simulink model "smo_pmsm"  (R2014a)
settings: Solver=ode45  StartTime=0.0  StopTime=3  RelTol=1e-3
PreLoadFcn:
  | parameter
InitFcn:
  | parameter
values from neighbouring files (symbols this model uses):
  R = 2e-3    (= 0.002)    [param.m]
undefined symbols (not defined in the file or in its folder): DiscIntNeverNeededParam, i_open_q, K, k_pll, ki_i, ki_pll, ki_v, kp_i, kp_pll, kp_v, L, sigbuilder_block, Threshold, TS, TS_time, upper, Vdc, wc, wc1, wc2
libraries: powerlib x4, AC6DriveInternalModels x1, simulink x1
Description:
  | parameter.m;
settings Model: SimulationMode=accelerator  Creator=jzj  LastModifiedBy=jzj
settings OptimizationCC: EfficientMapNaN2IntZero=off
settings HardwareCC: TargetLongLongMode=on  TargetIntDivRoundTo=Zero  TargetEndianess=LittleEndian  TargetHWDeviceType=MATLAB Host  ProdEqTarget=off
settings ModelReferenceCC: ModelDependencies=parameter.m;
settings CodeAppCC: MaxIdLength=128
settings GRTTargetCC: CombineOutputUpdateFcns=off  GRTInterface=on

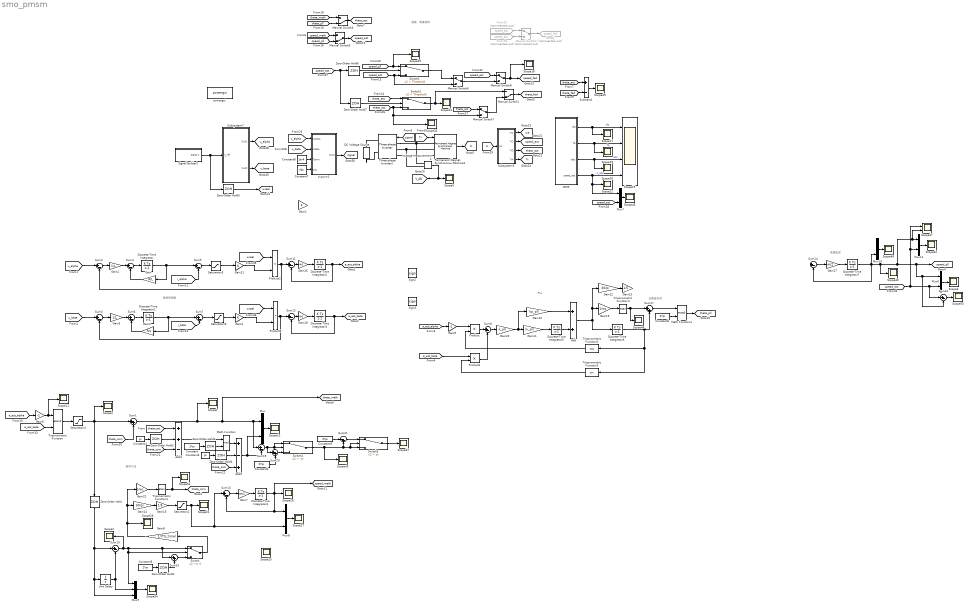
== system smo_pmsm ==
  note: 数学方法
  note: 滑模观测器
  note: 速度、角度选择
  note: 低通滤波
  note: PLL
  note: 加角度补偿
  Add : Sum
  Add1 : Sum  Inputs=++-
  Add2 : Sum  Inputs=+-+
  Constant{,2,5..6,9} (5 alike) : Constant  Value=2*pi
  Constant1 : Constant  Value=pi
  Constant3 : Constant  Value=pi
  Constant7 : Constant  Value=Vdc
  Constant8 : Constant  Value=1e-4
  DC Voltage Source : powerlib/Electrical Sources/DC Voltage Source  Amplitude=Vdc  Measurements=Voltage
  Discrete-Time Integrator{,1..3,6} (5 alike) : DiscreteIntegrator  SampleTime=-1  ICPrevOutput=DiscIntNeverNeededParam  ICPrevScaledInput=DiscIntNeverNeededParam
  Discrete-Time Integrator4 : DiscreteIntegrator  SampleTime=TS_time  ICPrevOutput=DiscIntNeverNeededParam  ICPrevScaledInput=DiscIntNeverNeededParam
  Discrete-Time Integrator5 : DiscreteIntegrator  InitialConditionSetting=State (most efficient)  SampleTime=-1  ICPrevOutput=DiscIntNeverNeededParam  ICPrevScaledInput=DiscIntNeverNeededParam
  Discrete-Time Integrator7 : DiscreteIntegrator  SampleTime=TS_time  ICPrevOutput=DiscIntNeverNeededParam  ICPrevScaledInput=DiscIntNeverNeededParam
  From15 : From  Commented=on  GotoTag=speed_act  TagVisibility=global
  From31 : From  Commented=on  GotoTag=speed_est  TagVisibility=global
  Gain : Gain  Gain=R/L
  Gain1 : Gain  Gain=K
  Gain10 : Gain  Gain=kp_pll
  Gain11 : Gain  Gain=ki_pll
  Gain12 : Gain  Gain=30/pi
  Gain13 : Gain  Gain=1/5
  Gain14 : Gain  Gain=30/pi
  Gain15 : Gain  Gain=1/5
  Gain16 : Gain  Gain=wc
  Gain17 : Gain  Gain=wc2
  Gain18 : Gain  Gain=wc
  Gain19 : Gain  Gain=1/wc
  Gain2 : Gain  Gain=1/L
  Gain20 : Gain  Gain=k_pll
  Gain21 : Gain  Gain=K
  Gain22 : Gain  Gain=2/wc
  Gain3 : Gain  Gain=R/L
  Gain4 : Gain  Gain=K
  Gain5 : Gain  Gain=1/L
  Gain6 : Gain  Gain=-1
  Gain7 : Gain  Gain=wc1
  Gain8 : Gain  Gain=1/(TS_time)
  Gain9 : Gain  Gain=-1
  Goto6 : Goto  Commented=on  GotoTag=speed_fed  TagVisibility=global
  Manual Switch1 : ManualSwitch  CurrentSetting=0
  Manual Switch2 : ManualSwitch  Commented=on
  Manual Switch3 : ManualSwitch  CurrentSetting=0
  Manual Switch5 : ManualSwitch  CurrentSetting=0
  Manual Switch6 : ManualSwitch
  Manual Switch7 : ManualSwitch
  Manual Switch8 : ManualSwitch
  Math Function : Math  Operator=mod  SaturateOnIntegerOverflow=on
  Math Function1 : Math  Operator=mod  SaturateOnIntegerOverflow=on
  Mux{,6..8,10..11} (6 alike) : Mux  Inputs=2
  Mux9 : Mux  Inputs=3
  Permanent Magnet Synchronous Machine1 : powerlib/Machines/Permanent Magnet Synchronous Machine  NbPhases=3  FluxDistribution=Sinusoidal  RotorType=Round  MechanicalLoad=Torque Tm  PresetModel=No  ShowDetailedParameters=on  MeasurementBus=off  Resistance=3  Inductance=0  dqInductances=[0.01,0.02]  La=0.0287  MachineConstant=Voltage Constant (V_peak L-L / krpm)  Flux=0.1654  VoltageCst=150  TorqueCst=1.2405  Flat=0  Mechanical=[0.001,0,5]  PolePairs=3  InitialConditions=[0,0, 0,0]  InitialConditions5ph=[0 0 0 0 0 0]  TsPowergui=0  TsBlock=-1  RefAngle=Aligned with phase A axis (original Park)
      link override From: GotoTag=tp24d3e2ed_e96a_4fb0_a076_5c3b1daf5e05
      settings: AttributesFormatString=\n
  Product{,1..3} (4 alike) : Product
  Saturation2 : Saturate  UpperLimit=5000  LowerLimit=-1000
  Saturation3 : Saturate  UpperLimit=upper  LowerLimit=-upper
  Saturation4 : Saturate  UpperLimit=pi  LowerLimit=-pi
  Saturation5 : Saturate  UpperLimit=upper  LowerLimit=-upper
  Scope{1..2,4..6,11,13,17..23,25..30,34,37,42..44,46,48..49,52,54..55} (31 alike) : Scope
      Scope1 settings: YMin=-700  YMax=700  SaveName=ScopeData7
      Scope11 settings: YMin=-700  YMax=700  SaveName=ScopeData25
      Scope13 settings: YMin=-700  YMax=700  SaveName=ScopeData32
      Scope17 settings: YMin=-700  YMax=700  SaveName=ScopeData18
      Scope18 settings: YMin=-700  YMax=700  SaveName=ScopeData35
      Scope19 settings: TimeRange=1.5  YMin=-700  YMax=700  SaveName=ScopeData19
      Scope2 settings: YMin=-700  YMax=700  SaveName=ScopeData10
      Scope20 settings: YMin=-0.04  YMax=0.04
      Scope21 settings: TimeRange=0.5  YMin=4000  YMax=4003  SaveName=ScopeData4
      Scope22 settings: YMin=-700  YMax=700  SaveName=ScopeData36
      Scope23 settings: YMin=-700  YMax=700  SaveName=ScopeData39
      Scope25 settings: YMin=-700  YMax=700  SaveName=ScopeData41
      Scope26 settings: YMin=-700  YMax=700  SaveName=ScopeData42
      Scope27 settings: YMin=-700  YMax=700  SaveName=ScopeData43
      Scope28 settings: YMin=-700  YMax=700  SaveName=ScopeData44
      Scope29 settings: YMin=-700  YMax=700  SaveName=ScopeData45
      Scope30 settings: YMin=-700  YMax=700  SaveName=ScopeData46
      Scope34 settings: YMin=-700  YMax=700  SaveName=ScopeData74
      Scope37 settings: YMin=-700  YMax=700  SaveName=ScopeData54
      Scope4 settings: YMin=-700  YMax=700  SaveName=ScopeData13
      Scope42 settings: YMin=-700  YMax=700  SaveName=ScopeData60
      Scope43 settings: YMin=-700  YMax=700  SaveName=ScopeData61
      Scope44 settings: YMin=-700  YMax=700  SaveName=ScopeData62
      Scope46 settings: TimeRange=0.5  YMin=0  YMax=600  SaveName=ScopeData63
      Scope48 settings: YMin=-700  YMax=700  SaveName=ScopeData73
      Scope49 settings: YMin=-700  YMax=700  SaveName=ScopeData80
      Scope5 settings: YMin=-700  YMax=700  SaveName=ScopeData78
      Scope52 settings: YMin=-700  YMax=700  SaveName=ScopeData77
      Scope54 settings: YMin=-700  YMax=700  SaveName=ScopeData81
      Scope55 settings: YMin=-700  YMax=700  SaveName=ScopeData85
      Scope6 settings: YMin=-700  YMax=700  SaveName=ScopeData14
  Scope15 : Scope  NumInputPorts=4
      settings: TimeRange=1.5  YMin=-17.5~-5~-80~-400  YMax=15~35~60~900  SaveName=ScopeData20
  Scope47 : Scope  NumInputPorts=2
      settings: YMin=-700~-5  YMax=700~5  SaveName=ScopeData76
  Sign2 : Signum
  Sign3 : Signum
  Signal Builder1 : Subsystem  Tag=STV Subsys  LoadFcn=sigbuilder_block('load');  StartFcn=sigbuilder_block('start');  StopFcn=sigbuilder_block('stop');  ClipboardFcn=sigbuilder_block('clipboard');  mask(Sigbuilder block){}
      mask help: Simulink:masks:SigbuilderBlock_MD
      mask init:
      | if ~strcmp(get_param(bdroot(gcbh),'SimulationStatus'),'stopped') tuvar = sigbuilder_block('maskInit'); end
      settings: CopyFcn=sigbuilder_block('copy');  DeleteFcn=sigbuilder_block('delete');  ModelCloseFcn=sigbuilder_block('modelClose');  PreSaveFcn=sigbuilder_block('preSave');  PauseFcn=sigbuilder_block('pause');  ContinueFcn=sigbuilder_block('continue');  NameChangeFcn=sigbuilder_block('namechange');  OpenFcn=sigbuilder_block('open',[6.75 -95.25 1138.5 566.25 ]);  CloseFcn=sigbuilder_block('close');
      mask Display: plot(0, 0, 100, 100,[2, 2, 32, 32, 2], [68, 8, 8, 68, 68],[32, 2], [38, 38], [32, 19, 2],[53, 60, 44], [32, 17, 17, 2],[16, 16, 31, 31]);txt = getActiveGroup(gcbh);text(2, 100, txt,'verticalAlignment', 'top');
  Subsystem3 : Subsystem
  Subsystem7 : Subsystem
  Subtract1 : Sum  Inputs=+-
  Sum{1,15,17,20} (4 alike) : Sum  Inputs=|++
  Sum{2..8,10..14,19,24} (14 alike) : Sum  Inputs=|+-
  Sum21 : Sum  Inputs=|-+
  Switch : Switch
  Switch1 : Switch  Criteria=u2 > Threshold  Threshold=Threshold
  Switch2 : Switch  Criteria=u2 > Threshold  Threshold=Threshold
  Switch4 : Switch  Criteria=u2 > Threshold  Threshold=-pi
  Switch5 : Switch  Criteria=u2 > Threshold  Threshold=pi
  Three-phase Inverter2 : AC6DriveInternalModels/Three-phase Inverter  Arms=3  SnubberResistance=5000  SnubberCapacitance=inf  Device=IGBT / Diodes  Ron=1e-3  Lon=0  ForwardVoltages=[0.8,0.8]  ForwardVoltage=0  GTOparameters=[0,0]  IGBTParameters=[1e-6,2e-6]  Measurements=All voltages and currents  converterType=Inverter  SourceFrequency=60  dqInductances=[8.5e-3,8.5e-3]  Flux=0.175  Resistance=0.2  p=4
  Trigonometric Function : Trigonometry  Operator=atan2
  Trigonometric Function1 : Trigonometry  Operator=atan
  Trigonometric Function2 : Trigonometry  Operator=cos
  Trigonometric Function3 : Trigonometry
  Trigonometric Function4 : Trigonometry  Operator=atan
  Unit Delay : UnitDelay  SampleTime=-1
  Voltage Measurement1 : powerlib/Measurements/Voltage Measurement  PhasorSimulation=off  OutputType=Complex  PSBequivalent=0
  Zero-Order Hold : ZeroOrderHold  SampleTime=TS_time
  Zero-Order Hold{1..7} (7 alike) : ZeroOrderHold  SampleTime=TS
  powergui : powerlib/powergui  Priority=1  SimulationMode=Discrete  SolverType=Tustin  SampleTime=1e-6  frequency=60  SPID=off  DisableSnubberDevices=off  DisableRonSwitches=off  DisableVfSwitches=off  SwTol=0  Interpol=off  DisplayEquations=off  Ts=100  methode=off  frequencyindice=0  Pbase=100e6  ErrMax=1e-4  Iterations=50  UnitsV=kV  UnitsW=MW  FunctionMessages=off  echomessages=off  HookPort=off  EnableUseOfTLC=off  x0status=blocks  RestoreLinks=warning  ResistiveCurrentMeasurement=off  Frange=[0:2:500]  Ylog=off  Xlog=on  ShowGrid=off  save=off  variable=ZData  structure=iabc1  ZoomFFT=off  StartTime=2.2  cycles=50  DisplayStyle=1  fundamental=200  FreqAxis=on  MaxFrequency=500  frequencyindicesteady=1  RmsSteady=1  display=off
  state : Subsystem
  svpwm1 : Subsystem
  tag scope: Tr=global, V_AB=global, e_est_alpha=global, e_est_beta=global, m=global, signal=global, speed_act=global, speed_est=global, speed_fed=global, speed_math=global, speed_pll=global, theta_act=global, theta_com=global, theta_est=global, theta_fed=global, theta_math=global, theta_pll=global, u_alpha=global, u_beta=global, we=global, wreal=global
  wires:
  Subsystem7/1(Out1) -> [u_alpha]
  Subsystem7/2(Out2) -> [u_beta]
  Constant8/1 -> svpwm1/3(Tpwm)
  Constant7/1 -> svpwm1/4(Vdc)
  svpwm1/1(Out1) -> [signal]
  [u_alpha] -> svpwm1/1(Valpha)
  [u_beta] -> svpwm1/2(Vbeta)
  [Tr] -> Permanent Magnet Synchronous Machine1/1
  Permanent Magnet Synchronous Machine1/1 -> [m]
  Voltage Measurement1/1 -> [V_AB], Scope5/1
  [m] -> Subsystem3/1(In1)
  Subsystem3/1(Tr1) -> [we]
  Subsystem3/2(Tr2) -> [speed_act]
  Subsystem3/3(Tr3) -> [theta_act]
  Subsystem3/4(Tr4) -> [Tr]
  state/1(idq) -> Scope17/1, Scope15/1  "idq"
  state/2(Te) -> Scope19/1, Scope15/2  "Te"
  state/3(iabc) -> Scope20/1, Scope15/3  "iabc"
  state/4(speed_obs) -> Mux7/1, Scope21/1, Scope15/4  "n_obs"
  Sum2/1 -> Gain2/1
  Sum4/1 -> Discrete-Time Integrator/1
  Gain/1 -> Sum4/2
  Discrete-Time Integrator/1 -> Sum5/1, Gain/1
  [i_alpha] -> Sum5/2
  Sum5/1 -> Saturation3/1
  Saturation3/1 -> Gain21/1
  Gain2/1 -> Sum4/1
  Sum6/1 -> Discrete-Time Integrator1/1
  Gain3/1 -> Sum6/2
  Discrete-Time Integrator1/1 -> Gain3/1, Sum7/1
  [i_beta] -> Sum7/2
  Sum7/1 -> Saturation5/1
  Saturation5/1 -> Gain4/1
  Gain5/1 -> Sum6/1
  Sum3/1 -> Gain5/1
  Gain6/1 -> Scope11/1, Trigonometric Function/1
  Product3/1 -> Sum3/2, Sum12/1
  Constant/1 -> Zero-Order Hold3/1
  Mux/1 -> Scope13/1
  [speed_act] -> Manual Switch6/2, Switch1/3
  [speed_pll] -> Scope29/1, Switch1/1
  [theta_est] -> Switch2/1
  [speed_est] -> Zero-Order Hold6/1, Zero-Order Hold7/1
  [theta_act] -> Switch2/3, Manual Switch7/2, Scope34/1
  Switch2/1 -> Scope23/1, Manual Switch1/1
  Trigonometric Function/1 -> Saturation4/1
  Gain8/1 -> Scope28/1, Gain14/1, Gain22/1
  Zero-Order Hold/1 -> Mux9/3, Unit Delay/1, Sum10/1
  Unit Delay/1 -> Sum10/2, Mux9/2
  Gain14/1 -> Gain15/1
  Sum11/1 -> Gain16/1
  Gain16/1 -> Discrete-Time Integrator2/1
  Discrete-Time Integrator2/1 -> [e_est_alpha], Sum11/2
  Sum12/1 -> Gain18/1
  Gain18/1 -> Discrete-Time Integrator3/1
  Discrete-Time Integrator3/1 -> [e_est_beta], Sum12/2
  Sum1/1 -> [theta_math], Sum19/1, Mux/1, Scope1/1
  Saturation4/1 -> Zero-Order Hold/1, Sum1/1, Scope4/1
  Gain15/1 -> Saturation2/1
  Mux9/1 -> Scope54/1
  Sum10/1 -> Scope2/1, Mux9/1, Switch/2, Sum15/1, Switch/1
  Sum15/1 -> Switch/3
  Switch/1 -> Gain8/1
  Sum13/1 -> Gain7/1
  Gain7/1 -> Discrete-Time Integrator4/1
  Discrete-Time Integrator4/1 -> [speed_math], Sum13/2, Mux8/1, Scope26/1
  Mux8/1 -> Scope27/1
  Manual Switch3/1 -> [theta_est]
  [e_est_alpha] -> Gain9/1
  Gain9/1 -> Product/1
  Product/1 -> Sum8/1
  Gain10/1 -> Add/1
  Discrete-Time Integrator5/1 -> Add/2
  Gain11/1 -> Discrete-Time Integrator5/1
  Sum8/1 -> Gain20/1
  Add/1 -> Gain19/1, Gain12/1, Discrete-Time Integrator6/1
  Discrete-Time Integrator6/1 -> Trigonometric Function3/1, Trigonometric Function2/1, Sum17/2
  Gain12/1 -> Gain13/1
  Trigonometric Function2/1 -> Product/2
  [e_est_beta] -> Product1/1
  Trigonometric Function3/1 -> Product1/2
  Product1/1 -> Sum8/2
  [theta_math] -> Manual Switch3/1
  [theta_pll] -> Manual Switch3/2
  Manual Switch5/1 -> [speed_est]
  [speed_math] -> Manual Switch5/1
  [speed_pll] -> Manual Switch5/2
  Sum14/1 -> Gain17/1
  Gain17/1 -> Discrete-Time Integrator7/1
  Discrete-Time Integrator7/1 -> Mux10/2, Sum14/2, Scope30/1, Scope47/2, Mux11/1, Sum24/2, Mux6/1, [speed_pll]
  Add1/1 -> Math Function/1
  Add2/1 -> Sum19/2, Mux/2
  Gain22/1 -> Trigonometric Function1/1
  Trigonometric Function1/1 -> Scope52/1, [theta_com]
  [theta_com] -> Sum1/2
  [theta_act] -> Add1/1
  Constant1/1 -> Zero-Order Hold2/1
  [theta_com] -> Add1/3
  Math Function/1 -> Add2/1
  Constant3/1 -> Zero-Order Hold4/1
  [theta_com] -> Add2/3
  Gain19/1 -> Trigonometric Function4/1
  Constant5/1 -> Zero-Order Hold1/1
  Zero-Order Hold2/1 -> Add1/2
  Zero-Order Hold3/1 -> Math Function/2
  Zero-Order Hold4/1 -> Add2/2
  Zero-Order Hold6/1 -> Switch1/2
  Zero-Order Hold7/1 -> Switch2/2
  Saturation2/1 -> Scope22/1, Sum13/1, Mux8/2
  Zero-Order Hold1/1 -> Sum15/2
  Gain20/1 -> Gain10/1, Gain11/1
  [speed_est] -> Mux7/2
  Mux7/1 -> Scope46/1
  Mux10/1 -> Scope48/1
  Signal Builder1/1(Signal 1) -> Zero-Order Hold5/1, Subsystem7/1(n_ref)
  [theta_act] -> Subtract1/1
  [theta_fed] -> Subtract1/2
  Subtract1/1 -> Scope49/1
  Manual Switch1/1 -> [theta_fed]
  From31/1 -> Manual Switch2/1
  From15/1 -> Manual Switch2/2
  Manual Switch2/1 -> Goto6/1
  Switch1/1 -> Manual Switch6/1
  [theta_act] -> Manual Switch7/1
  Manual Switch7/1 -> Manual Switch1/2
  Manual Switch6/1 -> Manual Switch8/2
  [speed_act] -> Manual Switch8/1
  Manual Switch8/1 -> Scope18/1, [speed_fed]
  [e_est_alpha] -> Gain6/1
  [e_est_beta] -> Trigonometric Function/2
  [u_alpha] -> Sum2/1
  [u_beta] -> Sum3/1
  [signal] -> Three-phase Inverter2/1
  Sum17/1 -> Math Function1/1
  Constant6/1 -> Math Function1/2
  Product2/1 -> Sum2/2, Sum11/1
  Sum19/1 -> Sum20/1, Switch4/1, Switch4/2
  Sum20/1 -> Switch4/3
  Constant2/1 -> Sum20/2
  Switch4/1 -> Scope43/1, Sum21/2, Switch5/2, Switch5/3
  Sum21/1 -> Switch5/1
  Constant9/1 -> Sum21/1
  Switch5/1 -> Scope37/1
  [speed_act] -> Scope47/1, Mux11/2, Sum24/1, Mux6/2
  Mux6/1 -> Scope6/1
  Mux11/1 -> Scope42/1
  Zero-Order Hold5/1 -> [wreal]
  Gain21/1 -> Product2/2
  Gain4/1 -> Product3/2
  [wreal] -> Product2/1
  [wreal] -> Product3/1
  Trigonometric Function4/1 -> Scope44/1, Sum17/1
  Sum24/1 -> Scope55/1
  Math Function1/1 -> [theta_pll]
  connections:
  Three-phase Inverter2/LConn1 -- Permanent Magnet Synchronous Machine1/LConn1 -- Voltage Measurement1/LConn1
  Voltage Measurement1/LConn2 -- Permanent Magnet Synchronous Machine1/LConn2 -- Three-phase Inverter2/LConn2
  Permanent Magnet Synchronous Machine1/LConn3 -- Three-phase Inverter2/LConn3
  DC Voltage Source/RConn1 -- Three-phase Inverter2/RConn1
  DC Voltage Source/LConn1 -- Three-phase Inverter2/RConn2

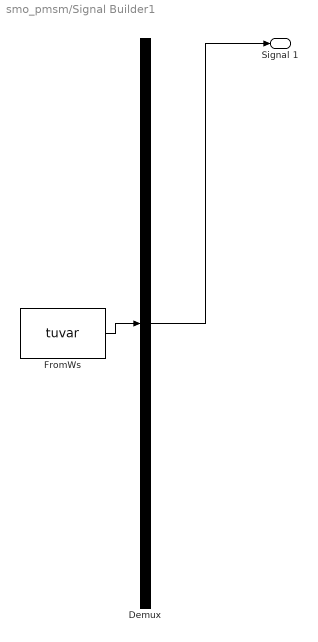
== system smo_pmsm/Signal Builder1 ==
  Demux : Demux  Tag=STV Demux  Outputs=1
  FromWs : FromWorkspace  Tag=STV FromWs  VariableName=tuvar  SampleTime=0
      SigBuilderData=|
      | common.afterFinalStr = 'Extrapolate'
      | common.sampleTime = 0
      | dataSet.timeRange = [0 10]
      | dataSet.name = 'Group 1'
      | sbobj.Groups.Name = 'Group 1'
      | sbobj.Groups.Signals.Name = 'Signal 1'
      | sbobj.Groups.Signals.XData = [0 0.5 4 6 10]
      | sbobj.Groups.Signals.YData = [0 1000 1000 1000 1000]
  Signal 1 : Outport  Tag=STV Outport
  wires:
  FromWs/1 -> Demux/1
  Demux/1 -> Signal 1/1

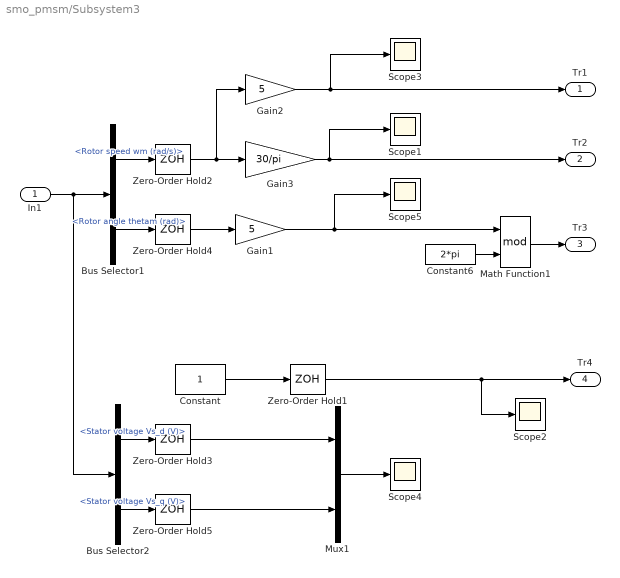
== system smo_pmsm/Subsystem3 ==
  In1 : Inport
  Bus Selector1 : BusSelector  OutputSignals=Rotor speed wm (rad/s),Rotor angle thetam (rad)
  Bus Selector2 : BusSelector  OutputSignals=Stator voltage Vs_d (V),Stator voltage Vs_q (V)
  Constant : Constant
  Constant6 : Constant  Value=2*pi
  Gain1 : Gain  Gain=5
  Gain2 : Gain  Gain=5
  Gain3 : Gain  Gain=30/pi
  Math Function1 : Math  Operator=mod  SaturateOnIntegerOverflow=on
  Mux1 : Mux  Inputs=2
  Scope{1..5} (5 alike) : Scope
      Scope1 settings: YMin=-500  YMax=700  SaveName=ScopeData9
      Scope2 settings: YMin=-25  YMax=400  SaveName=ScopeData149
      Scope3 settings: YMin=185.5  YMax=191.5  SaveName=ScopeData79
      Scope4 settings: YMin=-25  YMax=400  SaveName=ScopeData88
      Scope5 settings: YMin=195  YMax=202.5  SaveName=ScopeData90
  Zero-Order Hold{1..5} (5 alike) : ZeroOrderHold  SampleTime=TS
  Tr1 : Outport
  Tr2 : Outport  Port=2
  Tr3 : Outport  Port=3
  Tr4 : Outport  Port=4
  wires:
  Zero-Order Hold5/1 -> Mux1/2
  Zero-Order Hold3/1 -> Mux1/1
  Constant/1 -> Zero-Order Hold1/1
  In1/1 -> Bus Selector1/1, Bus Selector2/1
  Bus Selector1/1 -> Zero-Order Hold2/1  "<Rotor speed wm (rad/s)>"
  Bus Selector1/2 -> Zero-Order Hold4/1  "<Rotor angle thetam (rad)>"
  Zero-Order Hold2/1 -> Gain2/1, Gain3/1
  Zero-Order Hold4/1 -> Gain1/1
  Gain2/1 -> Tr1/1, Scope3/1
  Gain3/1 -> Scope1/1, Tr2/1
  Zero-Order Hold1/1 -> Scope2/1, Tr4/1
  Bus Selector2/1 -> Zero-Order Hold3/1  "<Stator voltage Vs_d (V)>"
  Bus Selector2/2 -> Zero-Order Hold5/1  "<Stator voltage Vs_q (V)>"
  Gain1/1 -> Math Function1/1, Scope5/1
  Mux1/1 -> Scope4/1
  Math Function1/1 -> Tr3/1
  Constant6/1 -> Math Function1/2

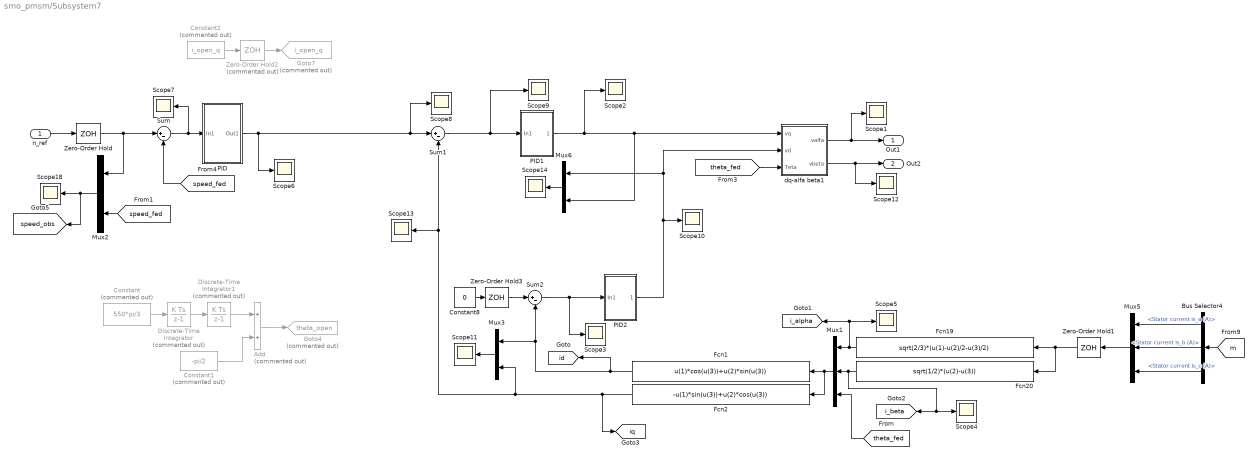
== system smo_pmsm/Subsystem7 ==
  n_ref : Inport
  Add : Sum  Commented=on
  Bus Selector4 : BusSelector  OutputSignals=Stator current is_a (A),Stator current is_b (A),Stator current is_c (A)
  Constant : Constant  Commented=on  Value=550*pi/3
  Constant1 : Constant  Commented=on  Value=-pi/2
  Constant2 : Constant  Commented=on  Value=i_open_q
  Constant8 : Constant  Value=0
  Discrete-Time Integrator : DiscreteIntegrator  Commented=on  InitialConditionSetting=State (most efficient)  SampleTime=-1  ICPrevOutput=DiscIntNeverNeededParam  ICPrevScaledInput=DiscIntNeverNeededParam
  Discrete-Time Integrator1 : DiscreteIntegrator  Commented=on  InitialConditionSetting=State (most efficient)  SampleTime=-1  ICPrevOutput=DiscIntNeverNeededParam  ICPrevScaledInput=DiscIntNeverNeededParam
  Fcn1 : Fcn  Expr=u(1)*cos(u(3))+u(2)*sin(u(3))
  Fcn19 : Fcn  Expr=sqrt(2/3)*(u(1)-u(2)/2-u(3)/2)
  Fcn2 : Fcn  Expr=-u(1)*sin(u(3))+u(2)*cos(u(3))
  Fcn20 : Fcn  Expr=sqrt(1/2)*(u(2)-u(3))
  Goto4 : Goto  Commented=on  GotoTag=theta_open  TagVisibility=global
  Goto7 : Goto  Commented=on  GotoTag=i_open_q  TagVisibility=global
  Mux1 : Mux  Inputs=3
  Mux2 : Mux  Inputs=2
  Mux3 : Mux  Inputs=2
  Mux5 : Mux  Inputs=3
  Mux6 : Mux  Inputs=2
  PID : Subsystem
  PID1 : Subsystem
  PID2 : Subsystem
  Scope{1..14,18} (15 alike) : Scope
      Scope1 settings: SaveName=ScopeData37
      Scope10 settings: SaveName=ScopeData30
      Scope11 settings: TimeRange=1.7  YMin=-15  YMax=17.5  SaveName=ScopeData71
      Scope12 settings: SaveName=ScopeData17
      Scope13 settings: SaveName=ScopeData75
      Scope14 settings: TimeRange=1.7  YMin=-15  YMax=17.5  SaveName=ScopeData106
      Scope18 settings: TimeRange=0.01073731461302402  YMin=996.9949713569969  YMax=1006.526183941498  SaveName=ScopeData21
      Scope2 settings: SaveName=ScopeData22
      Scope3 settings: SaveName=ScopeData23
      Scope4 settings: SaveName=ScopeData47
      Scope5 settings: SaveName=ScopeData48
      Scope6 settings: SaveName=ScopeData38
      Scope7 settings: SaveName=ScopeData26
      Scope8 settings: SaveName=ScopeData28
      Scope9 settings: SaveName=ScopeData29
  Sum : Sum  Inputs=|+-
  Sum1 : Sum  Inputs=|+-
  Sum2 : Sum  Inputs=|+-
  Zero-Order Hold : ZeroOrderHold  SampleTime=TS
  Zero-Order Hold1 : ZeroOrderHold  SampleTime=TS
  Zero-Order Hold2 : ZeroOrderHold  Commented=on  SampleTime=TS
  Zero-Order Hold3 : ZeroOrderHold  SampleTime=TS
  dq-alfa beta1 : Subsystem
  Out1 : Outport
  Out2 : Outport  Port=2
  tag scope: i_alpha=global, i_beta=global, id=global, iq=global, speed_obs=global
  wires:
  Sum1/1 -> PID1/1(In1), Scope9/1
  Sum2/1 -> Scope3/1, PID2/1(In1)
  Mux2/1 -> [speed_obs], Scope18/1
  Sum/1 -> PID/1(In1), Scope7/1
  Constant8/1 -> Zero-Order Hold3/1
  Zero-Order Hold3/1 -> Sum2/1
  [speed_fed] -> Mux2/2
  Zero-Order Hold/1 -> Sum/1, Mux2/1
  n_ref/1 -> Zero-Order Hold/1
  Mux3/1 -> Scope11/1
  [speed_fed] -> Sum/2
  dq-alfa beta1/1(valfa) -> Out1/1, Scope1/1
  dq-alfa beta1/2(vbeta) -> Scope12/1, Out2/1
  Fcn1/1 -> Mux3/1, Sum2/2, [id]
  Fcn2/1 -> [iq], Scope13/1, Sum1/2, Mux3/2
  Mux6/1 -> Scope14/1
  [m] -> Bus Selector4/1
  Bus Selector4/2 -> Mux5/2  "<Stator current is_b (A)>"
  Bus Selector4/3 -> Mux5/3  "<Stator current is_c (A)>"
  Bus Selector4/1 -> Mux5/1  "<Stator current is_a (A)>"
  Mux5/1 -> Zero-Order Hold1/1
  Fcn19/1 -> Scope5/1, [i_alpha], Mux1/1
  Fcn20/1 -> [i_beta], Scope4/1, Mux1/2
  [theta_fed] -> Mux1/3
  Mux1/1 -> Fcn2/1, Fcn1/1
  Zero-Order Hold1/1 -> Fcn20/1, Fcn19/1
  PID1/1(Out1) -> dq-alfa beta1/1(vq), Mux6/2, Scope2/1
  PID2/1(Out1) -> Scope10/1, dq-alfa beta1/2(vd), Mux6/1
  Constant/1 -> Discrete-Time Integrator/1
  Discrete-Time Integrator/1 -> Discrete-Time Integrator1/1
  Discrete-Time Integrator1/1 -> Add/1
  Constant1/1 -> Add/2
  Add/1 -> Goto4/1
  Constant2/1 -> Zero-Order Hold2/1
  Zero-Order Hold2/1 -> Goto7/1
  [theta_fed] -> dq-alfa beta1/3(Teta)
  PID/1(Out1) -> Scope6/1, Scope8/1, Sum1/1

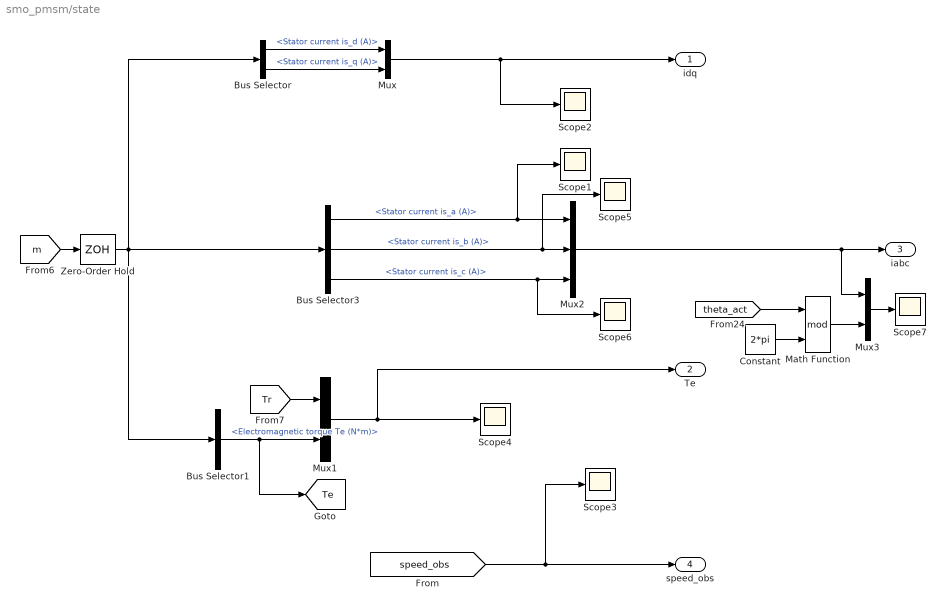
== system smo_pmsm/state ==
  Bus Selector : BusSelector  OutputSignals=Stator current is_d (A),Stator current is_q (A)
  Bus Selector1 : BusSelector  OutputSignals=Electromagnetic torque Te (N*m)
  Bus Selector3 : BusSelector  OutputSignals=Stator current is_a (A),Stator current is_b (A),Stator current is_c (A)
  Constant : Constant  Value=2*pi
  Math Function : Math  Operator=mod  SaturateOnIntegerOverflow=on
  Mux : Mux  Inputs=2
  Mux1 : Mux  Inputs=2
  Mux2 : Mux  Inputs=3
  Mux3 : Mux  Inputs=2
  Scope{1..7} (7 alike) : Scope
      Scope1 settings: TimeRange=0.7000000000000001  YMin=-4  YMax=8  SaveName=iabc
      Scope2 settings: TimeRange=0.7000000000000001  YMin=-2  YMax=18  SaveName=iabc1
      Scope3 settings: TimeRange=0.7000000000000001  YMin=1700  YMax=1712  SaveName=iabc2
      Scope4 settings: TimeRange=0.7000000000000001  YMin=-4  YMax=8  SaveName=iabc3
      Scope5 settings: TimeRange=0.7000000000000001  YMin=-4  YMax=8  SaveName=iabc4
      Scope6 settings: TimeRange=0.7000000000000001  YMin=-4  YMax=8  SaveName=iabc5
      Scope7 settings: TimeRange=0.7000000000000001  YMin=-4  YMax=8  SaveName=iabc6
  Zero-Order Hold : ZeroOrderHold  SampleTime=TS
  idq : Outport
  Te : Outport  Port=2
  iabc : Outport  Port=3
  speed_obs : Outport  Port=4
  tag scope: Te=global
  wires:
  Bus Selector/1 -> Mux/1  "<Stator current is_d (A)>"
  Bus Selector/2 -> Mux/2  "<Stator current is_q (A)>"
  Bus Selector3/1 -> Mux2/1, Scope1/1  "<Stator current is_a (A)>"
  Bus Selector3/3 -> Scope6/1, Mux2/3  "<Stator current is_c (A)>"
  Bus Selector3/2 -> Scope5/1, Mux2/2  "<Stator current is_b (A)>"
  Bus Selector1/1 -> [Te], Mux1/2  "<Electromagnetic torque Te (N*m)>"
  [m] -> Zero-Order Hold/1
  [Tr] -> Mux1/1
  Mux/1 -> Scope2/1, idq/1
  Zero-Order Hold/1 -> Bus Selector/1, Bus Selector1/1, Bus Selector3/1
  Mux2/1 -> Mux3/1, iabc/1
  [speed_obs] -> Scope3/1, speed_obs/1
  Mux1/1 -> Scope4/1, Te/1
  [theta_act] -> Math Function/1
  Constant/1 -> Math Function/2
  Math Function/1 -> Mux3/2
  Mux3/1 -> Scope7/1

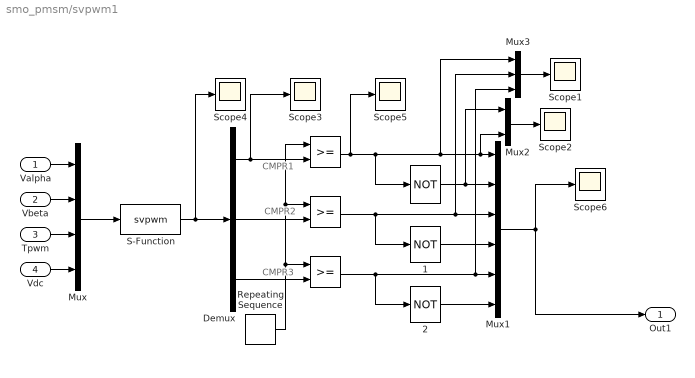
== system smo_pmsm/svpwm1 ==
  note: CMPR1
  note: CMPR2
  note: CMPR3
  Valpha : Inport
  Vbeta : Inport  Port=2
  Tpwm : Inport  Port=3
  Vdc : Inport  Port=4
  " " : RelationalOperator  ZeroCross=off
  "  " : RelationalOperator  OutDataTypeStr=boolean
  "   " : RelationalOperator  OutDataTypeStr=boolean
  "    " : Logic  Operator=NOT  Inputs=1  AllPortsSameDT=off  OutDataTypeStr=boolean
  "    1" : Logic  Operator=NOT  Inputs=1  AllPortsSameDT=off  OutDataTypeStr=boolean
  "    2" : Logic  Operator=NOT  Inputs=1  AllPortsSameDT=off  OutDataTypeStr=boolean
  Demux : Demux  Outputs=3
  Mux : Mux
  Mux1 : Mux  Inputs=6
  Mux2 : Mux  Inputs=2
  Mux3 : Mux  Inputs=3
  Repeating Sequence : simulink/Sources/Repeating Sequence  rep_seq_t=[0 0.00005 0.0001]  rep_seq_y=[0 0.00005 0]
  S-Function : S-Function  FunctionName=svpwm  EnableBusSupport=off
  Scope{1..6} (6 alike) : Scope
      Scope1 settings: TimeRange=1  YMin=-1  YMax=2  SaveName=ScopeData3
      Scope2 settings: TimeRange=0.2  YMin=-2.5e-006  YMax=5.25e-005  SaveName=ScopeData5
      Scope3 settings: TimeRange=0.2  YMin=-2.5e-006  YMax=5.25e-005
      Scope4 settings: TimeRange=0.2  YMin=-2.5e-006  YMax=5.25e-005  SaveName=ScopeData6
      Scope5 settings: TimeRange=0.2  YMin=-2.5e-006  YMax=5.25e-005  SaveName=ScopeData2
      Scope6 settings: TimeRange=0.2  YMin=-2.5e-006  YMax=5.25e-005  SaveName=ScopeData8
  Out1 : Outport
  wires:
  Demux/1 -> " "/2, Scope3/1
  Demux/2 -> "  "/2
  Demux/3 -> "   "/2
  "   "/1 -> "    2"/1, Mux1/5, Mux3/3
  "    "/1 -> Mux1/2, Mux2/1
  " "/1 -> Mux1/1, Mux2/2, Mux3/1, "    "/1, Scope5/1
  "  "/1 -> "    1"/1, Mux1/3, Mux3/2
  "    1"/1 -> Mux1/4
  "    2"/1 -> Mux1/6
  Repeating Sequence/1 -> "  "/1, " "/1, "   "/1
  S-Function/1 -> Demux/1, Scope4/1
  Valpha/1 -> Mux/1
  Vbeta/1 -> Mux/2
  Tpwm/1 -> Mux/3
  Vdc/1 -> Mux/4
  Mux3/1 -> Scope1/1
  Mux/1 -> S-Function/1
  Mux1/1 -> Out1/1, Scope6/1
  Mux2/1 -> Scope2/1

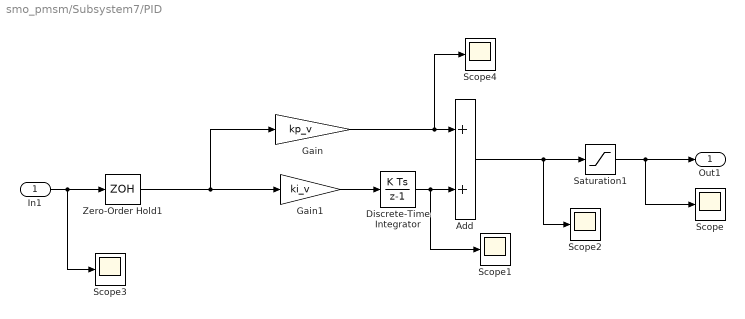
== system smo_pmsm/Subsystem7/PID ==
  In1 : Inport
  Add : Sum
  Discrete-Time Integrator : DiscreteIntegrator  InitialConditionSetting=State (most efficient)  SampleTime=-1  ICPrevOutput=DiscIntNeverNeededParam  ICPrevScaledInput=DiscIntNeverNeededParam
  Gain : Gain  Gain=kp_v
  Gain1 : Gain  Gain=ki_v
  Saturation1 : Saturate  UpperLimit=3  LowerLimit=-2
  Scope{,1..4} (5 alike) : Scope
      Scope settings: SaveName=ScopeData12
      Scope1 settings: SaveName=ScopeData27
      Scope2 settings: SaveName=ScopeData68
      Scope3 settings: SaveName=ScopeData69
      Scope4 settings: SaveName=ScopeData87
  Zero-Order Hold1 : ZeroOrderHold  SampleTime=TS
  Out1 : Outport
  wires:
  In1/1 -> Scope3/1, Zero-Order Hold1/1
  Gain/1 -> Scope4/1, Add/1
  Discrete-Time Integrator/1 -> Scope1/1, Add/2
  Add/1 -> Saturation1/1, Scope2/1
  Gain1/1 -> Discrete-Time Integrator/1
  Zero-Order Hold1/1 -> Gain/1, Gain1/1
  Saturation1/1 -> Out1/1, Scope/1

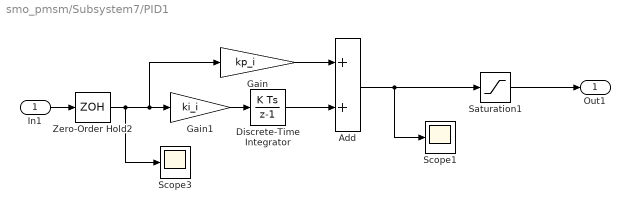
== system smo_pmsm/Subsystem7/PID1 ==
  In1 : Inport
  Add : Sum
  Discrete-Time Integrator : DiscreteIntegrator  InitialConditionSetting=State (most efficient)  SampleTime=-1  ICPrevOutput=DiscIntNeverNeededParam  ICPrevScaledInput=DiscIntNeverNeededParam
  Gain : Gain  Gain=kp_i
  Gain1 : Gain  Gain=ki_i
  Saturation1 : Saturate  UpperLimit=500  LowerLimit=-500
  Scope1 : Scope
      settings: SaveName=ScopeData64
  Scope3 : Scope
      settings: SaveName=ScopeData65
  Zero-Order Hold2 : ZeroOrderHold  SampleTime=TS
  Out1 : Outport
  wires:
  Add/1 -> Saturation1/1, Scope1/1
  Discrete-Time Integrator/1 -> Add/2
  Gain/1 -> Add/1
  Gain1/1 -> Discrete-Time Integrator/1
  In1/1 -> Zero-Order Hold2/1
  Zero-Order Hold2/1 -> Scope3/1, Gain/1, Gain1/1
  Saturation1/1 -> Out1/1

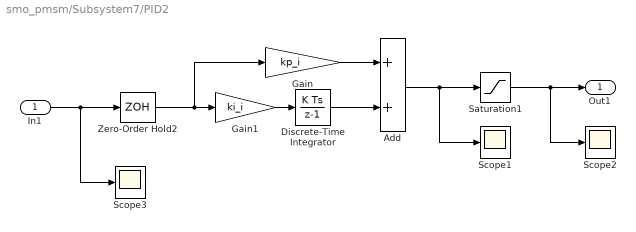
== system smo_pmsm/Subsystem7/PID2 ==
  In1 : Inport
  Add : Sum
  Discrete-Time Integrator : DiscreteIntegrator  InitialConditionSetting=State (most efficient)  SampleTime=-1  ICPrevOutput=DiscIntNeverNeededParam  ICPrevScaledInput=DiscIntNeverNeededParam
  Gain : Gain  Gain=kp_i
  Gain1 : Gain  Gain=ki_i
  Saturation1 : Saturate  UpperLimit=500  LowerLimit=-500
  Scope1 : Scope
      settings: YMin=-185  YMax=-115  SaveName=ScopeData67
  Scope2 : Scope
      settings: SaveName=ScopeData66
  Scope3 : Scope
      settings: SaveName=ScopeData70
  Zero-Order Hold2 : ZeroOrderHold  SampleTime=TS
  Out1 : Outport
  wires:
  Zero-Order Hold2/1 -> Gain1/1, Gain/1
  In1/1 -> Scope3/1, Zero-Order Hold2/1
  Gain1/1 -> Discrete-Time Integrator/1
  Gain/1 -> Add/1
  Discrete-Time Integrator/1 -> Add/2
  Add/1 -> Saturation1/1, Scope1/1
  Saturation1/1 -> Scope2/1, Out1/1

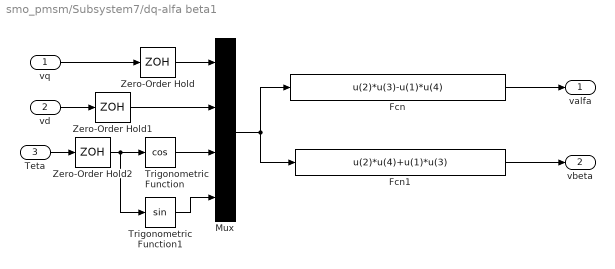
== system smo_pmsm/Subsystem7/dq-alfa beta1 ==
  vq : Inport
  vd : Inport  Port=2
  Teta : Inport  Port=3
  Fcn : Fcn  Expr=u(2)*u(3)-u(1)*u(4)
  Fcn1 : Fcn  Expr=u(2)*u(4)+u(1)*u(3)
  Mux : Mux
  Trigonometric Function : Trigonometry  Operator=cos
  Trigonometric Function1 : Trigonometry
  Zero-Order Hold : ZeroOrderHold  SampleTime=TS
  Zero-Order Hold1 : ZeroOrderHold  SampleTime=TS
  Zero-Order Hold2 : ZeroOrderHold  SampleTime=TS
  valfa : Outport
  vbeta : Outport  Port=2
  wires:
  Mux/1 -> Fcn/1, Fcn1/1
  Fcn/1 -> valfa/1
  Fcn1/1 -> vbeta/1
  Trigonometric Function/1 -> Mux/3
  Trigonometric Function1/1 -> Mux/4
  vq/1 -> Zero-Order Hold/1
  Zero-Order Hold/1 -> Mux/1
  vd/1 -> Zero-Order Hold1/1
  Zero-Order Hold1/1 -> Mux/2
  Teta/1 -> Zero-Order Hold2/1
  Zero-Order Hold2/1 -> Trigonometric Function/1, Trigonometric Function1/1
